simulink model "bouclage_echec"  (R2018b)
settings: Solver=FixedStepAuto  StartTime=0.0  StopTime=10.0  FixedStep=1e-5  RelTol=1e-3
model workspace (MAT data in the model file):
  Jb = 0.0059
  Jp = 0.0021
  Ks = 1.61
  N = 70
  R = 2.6
  g = 9.81
  h = 0.06
  m = 0.403
  phi = 0.00767
values from neighbouring files (symbols this model uses):
  A = [0 0                   1                   0 ... (first row only)    [load_param.m]
  B = [0            0 ... (first row only)    [load_param.m]
settings Model: Creator=pac  LastModifiedBy=pac

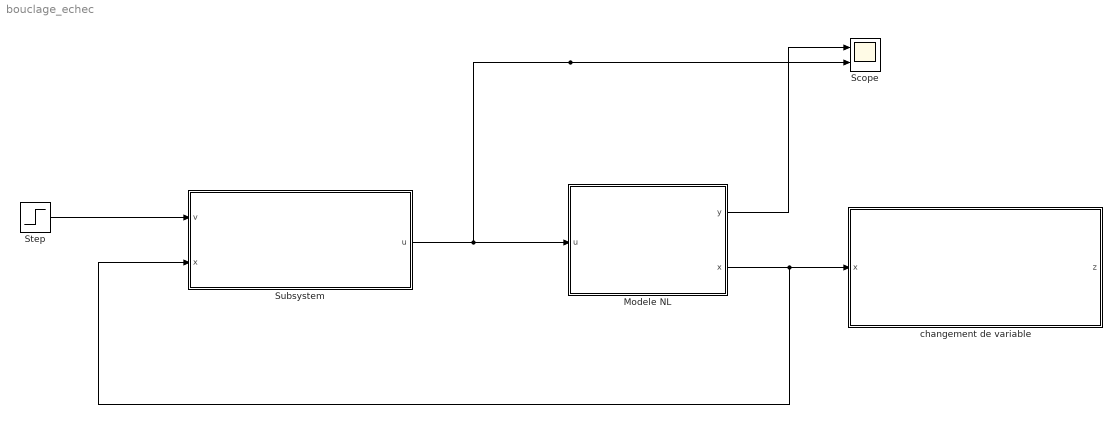
== system bouclage_echec ==
  Modele NL : Subsystem
  Scope : Scope  NumInputPorts=2
  Step : Step  SampleTime=0
  Subsystem : Subsystem
  changement de variable : Subsystem
  wires:
  Modele NL/1(y) -> Scope/1
  Modele NL/2(x) -> Subsystem/2(x), changement de variable/1(x)
  Subsystem/1(u) -> Scope/2, Modele NL/1(u)
  Step/1 -> Subsystem/1(v)

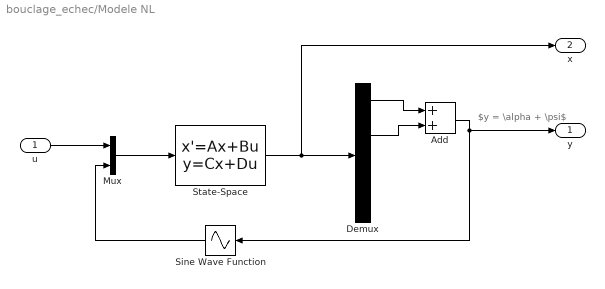
== system bouclage_echec/Modele NL ==
  note: $y = \alpha + \psi$
  u : Inport
  Add : Sum
  Demux : Demux
  Mux : Mux  Inputs=2
  Sine Wave Function : Sin  TimeSource=Use external signal  Amplitude=N*phi/(R*Jp)  SampleTime=0
  State-Space : StateSpace  A=A  B=B  C=[1 0 0 0 ; 0 1 0 0 ;0 0 1 0; 0 0 0 1]  D=[0 0; 0 0; 0 0; 0 0]  InitialCondition=0
  y : Outport
  x : Outport  Port=2
  wires:
  Demux/2 -> Add/2
  Mux/1 -> State-Space/1
  Sine Wave Function/1 -> Mux/2
  State-Space/1 -> x/1, Demux/1
  Add/1 -> y/1, Sine Wave Function/1
  u/1 -> Mux/1
  Demux/1 -> Add/1

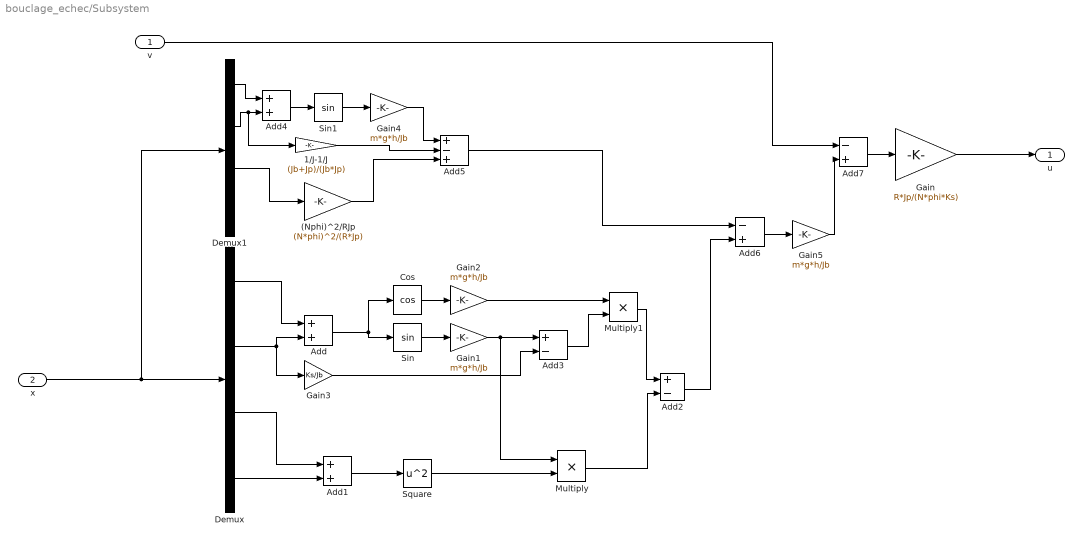
== system bouclage_echec/Subsystem ==
  v : Inport
  x : Inport  Port=2
  "(Nphi)^2/RJp " : Gain  Gain=(N*phi)^2/(R*Jp)
  1/J-1/J : Gain  Gain=(Jb+Jp)/(Jb*Jp)
  Add : Sum
  Add1 : Sum
  Add2 : Sum  Inputs=+-
  Add3 : Sum  Inputs=+-
  Add4 : Sum
  Add5 : Sum  Inputs=+-+
  Add6 : Sum  Inputs=-+
  Add7 : Sum  Inputs=-+
  Cos : Trigonometry  Operator=cos
  Demux : Demux
  Demux1 : Demux
  Gain : Gain  Gain=R*Jp/(N*phi*Ks)
  Gain{1..2,4..5} (4 alike) : Gain  Gain=m*g*h/Jb
  Gain3 : Gain  Gain=Ks/Jb
  Multiply : Product
  Multiply1 : Product
  Sin : Trigonometry
  Sin1 : Trigonometry
  Square : Math  Operator=square  SaturateOnIntegerOverflow=on
  u : Outport
  wires:
  Add3/1 -> Multiply1/2
  Gain3/1 -> Add3/2
  Add4/1 -> Sin1/1
  Add1/1 -> Square/1
  Add2/1 -> Add6/2
  Multiply1/1 -> Add2/1
  Add5/1 -> Add6/1
  Sin/1 -> Gain1/1
  Multiply/1 -> Add2/2
  Demux1/2 -> 1/J-1/J/1, Add4/2
  Demux/2 -> Add/2, Gain3/1
  Demux1/3 -> "(Nphi)^2/RJp "/1
  Demux/4 -> Add1/2
  "(Nphi)^2/RJp "/1 -> Add5/3
  Demux/3 -> Add1/1
  x/1 -> Demux/1, Demux1/1
  Gain1/1 -> Add3/1, Multiply/1
  Sin1/1 -> Gain4/1
  1/J-1/J/1 -> Add5/2
  Demux/1 -> Add/1
  Gain2/1 -> Multiply1/1
  Demux1/1 -> Add4/1
  Square/1 -> Multiply/2
  Add/1 -> Cos/1, Sin/1
  Gain4/1 -> Add5/1
  Cos/1 -> Gain2/1
  Gain/1 -> u/1
  v/1 -> Add7/1
  Add7/1 -> Gain/1
  Add6/1 -> Gain5/1
  Gain5/1 -> Add7/2

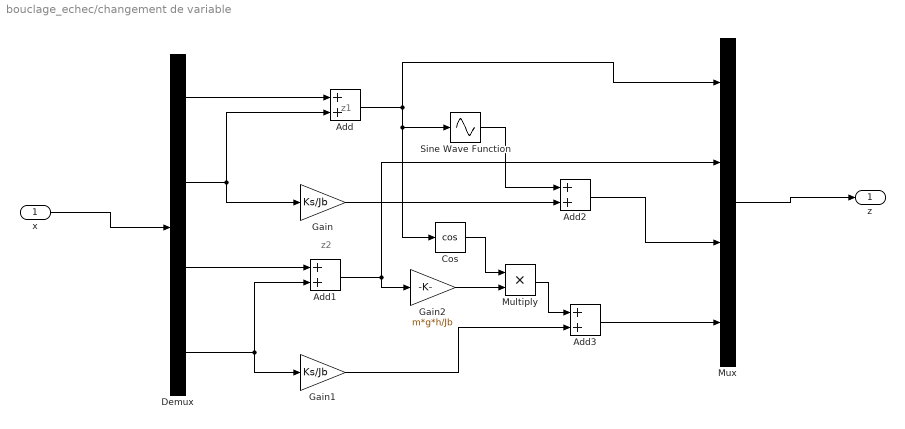
== system bouclage_echec/changement de variable ==
  note: z2
  note: z1
  x : Inport
  Add{,1..3} (4 alike) : Sum
  Cos : Trigonometry  Operator=cos
  Demux : Demux
  Gain : Gain  Gain=Ks/Jb
  Gain1 : Gain  Gain=Ks/Jb
  Gain2 : Gain  Gain=m*g*h/Jb
  Multiply : Product
  Mux : Mux
  Sine Wave Function : Sin  TimeSource=Use external signal  Amplitude=m*g*h/Jb  SampleTime=0
  z : Outport
  wires:
  Mux/1 -> z/1
  Multiply/1 -> Add3/1
  Gain1/1 -> Add3/2
  Demux/1 -> Add/1
  Cos/1 -> Multiply/1
  Add2/1 -> Mux/3
  Add/1 -> Cos/1, Sine Wave Function/1, Mux/1
  Demux/3 -> Add1/1
  Gain2/1 -> Multiply/2
  Demux/4 -> Add1/2, Gain1/1
  Sine Wave Function/1 -> Add2/1
  Demux/2 -> Add/2, Gain/1
  Add1/1 -> Mux/2, Gain2/1
  Add3/1 -> Mux/4
  x/1 -> Demux/1
  Gain/1 -> Add2/2
